simulink model "FCS_MPC_3Phase_SPMSM_TEST1"  (R2022a)
settings: Solver=ode23t  StartTime=0.0  StopTime=0.2  RelTol=1e-3  AbsTol=1e-3  EnableMultiTasking=on
values from neighbouring files (symbols this model uses):
  f_c = 100000    [FCS_MPC_3Phase_SPMSM_Params.m]
  Ld = 0.0003    [FCS_MPC_3Phase_SPMSM_Params.m]
  Lq = 0.0003    [FCS_MPC_3Phase_SPMSM_Params.m]
  np = 4    [FCS_MPC_3Phase_SPMSM_Params.m]
  psiPM = 0.0075    [FCS_MPC_3Phase_SPMSM_Params.m]
  R = 0.085    [FCS_MPC_3Phase_SPMSM_Params.m]
  T_50MHz = 1/f_50MHz    (= 2e-08)    [FCS_MPC_3Phase_SPMSM_Params.m]
  u_dc = 24    [FCS_MPC_3Phase_SPMSM_Params.m]
libraries: ee_lib x22, nesl_utility x22, fl_lib x21, simulink x7
(part 1 of 2)
settings Model: Creator=Michael Hoerner  LastModifiedBy=Andre Merx
settings SolverCC: AutoScaleAbsTol=off  AlgebraicLoopSolver=TrustRegion  DecoupledContinuousIntegration=on  MinimalZcImpactIntegration=on
settings DataIOCC: LimitDataPoints=on  MaxDataPoints=10000  ReturnWorkspaceOutputs=off
settings OptimizationCC: BlockReduction=off  ConditionallyExecuteInputs=off  DefaultParameterBehavior=Inlined  StrengthReduction=on  PassReuseOutputArgsAs=Individual arguments  OptimizeBlockOrder=speed  OptimizationPriority=Speed  OptimizationCustomize=off  MultiThreadedLoops=on  EfficientTunableParamExpr=on
settings DebuggingCC: AlgebraicLoopMsg=error  ParameterTunabilityLossMsg=error  UnconnectedInputMsg=warning  UnconnectedOutputMsg=warning  UnconnectedLineMsg=warning  AllowSymbolicDim=off  SFUnexpectedBacktrackingDiag=warning  SFNoUnconditionalDefaultTransitionDiag=warning  SFExecutionAtInitializationDiag=none  SFMachineParentedDataDiag=warning  ArithmeticOperatorsInVariantConditions=warning
settings HardwareCC: ProdBitPerPointer=32  ProdBitPerSizeT=32  ProdBitPerPtrDiffT=32  ProdLargestAtomicFloat=None  ProdIntDivRoundTo=Undefined  ProdEndianess=Unspecified  ProdWordSize=32  ProdHWDeviceType=ASIC/FPGA->ASIC/FPGA  TargetBitPerPointer=64  TargetBitPerSizeT=64  TargetBitPerPtrDiffT=64  TargetLongLongMode=on  TargetIntDivRoundTo=Zero  TargetEndianess=LittleEndian  TargetWordSize=64  TargetHWDeviceType=Custom Processor->MATLAB Host Computer  ProdEqTarget=off
settings SFSimCC: SimUseLocalCustomCode=off  MATLABDynamicMemAlloc=off  CustomCodeUndefinedFunction=UseInterfaceOnly
settings RTWCC: SystemTargetFile=ert.tlc  TemplateMakefile=ert_default_tmf  GenerateReport=on  RTWUseLocalCustomCode=off  IncludeHyperlinkInReport=on  LaunchReport=on  GenerateTraceInfo=on  GenerateTraceReport=on  GenerateTraceReportSl=on  GenerateTraceReportSf=on  GenerateTraceReportEml=on  DLArmComputeVersion=19.05
settings CodeAppCC: ForceParamTrailComments=on  IgnoreCustomStorageClasses=off  OperatorAnnotations=on  SimulinkDataObjDesc=on  SFDataObjDesc=on  InsertBlockDesc=on
settings ERTTargetCC: CodeReplacementLibrary=TI C28x with C99 extensions  GenerateSampleERTMain=on  CodeInterfacePackaging=Reusable function  MultiInstanceErrorCode=Warning  ERTCustomFileTemplate=example_file_process.tlc  ERTFilePackagingFormat=Compact
settings ConfigComp: CovMetricSettings=dw  CovSaveCumulativeToWorkspaceVar=on  CovSaveSingleToWorkspaceVar=on  CovExternalEMLEnable=off  CovSFcnEnable=off
settings SimscapeCC: SimscapeLogDataHistory=10000

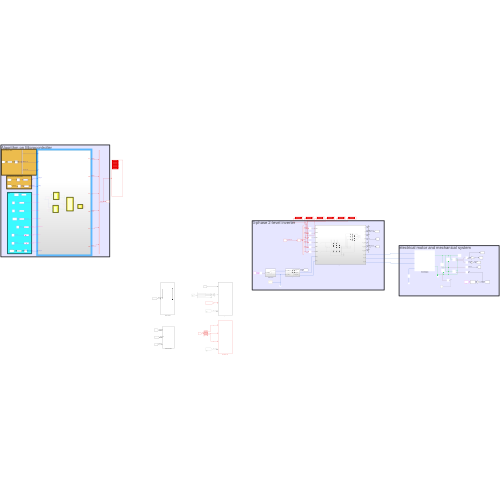
[thumbnail: Simulink's stored preview of the top-level diagram]
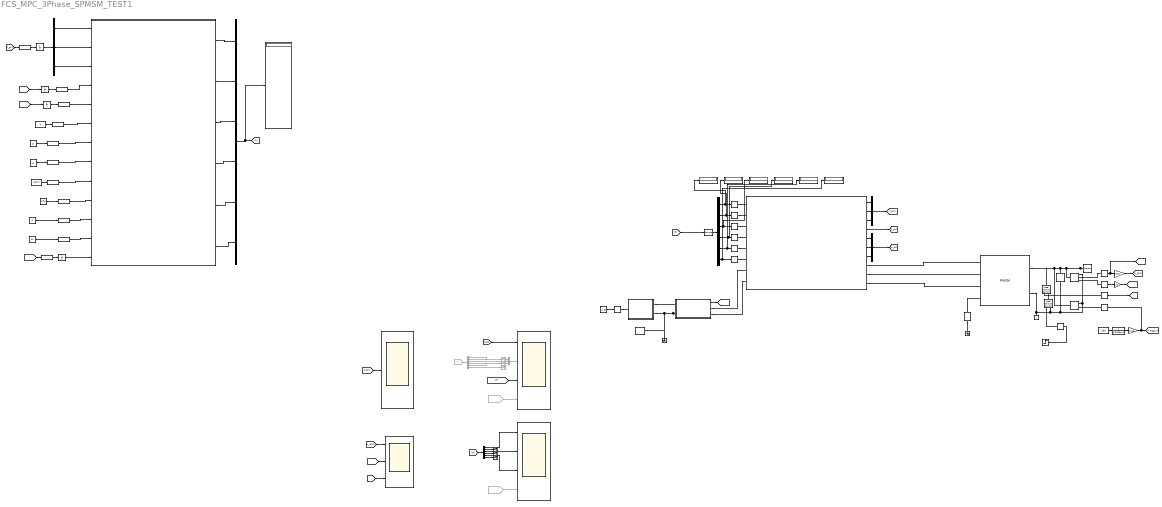
== system FCS_MPC_3Phase_SPMSM_TEST1 ==
  note: electrical motor and mechanical system
  note: 3-phase 2-level inverter
  note: Algorithm on Microcontroller
  note: AXI
  note: Von IP-Core IncreEncoder
  note: Von IP-Core ADC
  3ph_Inverter : Subsystem
  Constant : Constant  Value=Ld
  Constant1 : Constant  Value=R
  Constant11 : Constant  Value=1/f_c
  Constant6 : Constant  Value=u_dc
  Constant8 : Constant  Value=psiPM
  Constant9 : Constant  Value=Lq
  DC_link : Subsystem
  Data Type Conversion : DataTypeConversion  OutDataTypeStr=double  SaturateOnIntegerOverflow=off  RndMeth=Floor
  Data Type Conversion{4,6,10..11} (4 alike) : DataTypeConversion  OutDataTypeStr=fixdt(1,24,20)  SaturateOnIntegerOverflow=off  RndMeth=Floor
  Data Type Conversion{2,5,7..9,24} (6 alike) : DataTypeConversion  OutDataTypeStr=fixdt(1,18,11)  SaturateOnIntegerOverflow=off  RndMeth=Floor
  Data Type Conversion3 : DataTypeConversion  OutDataTypeStr=fixdt(1,24,11)  SaturateOnIntegerOverflow=off  RndMeth=Floor
  Demux : Demux  Outputs=3
  Demux2 : Demux  Outputs=6
  Demux3 : Demux  Commented=on  Outputs=6
  Demux4 : Demux  Outputs=6
  Display{1..7} (7 alike) : Display
  Electrical Reference1 : fl_lib/Electrical/Electrical Elements/Electrical Reference
      settings: SourceProductBaseCode=PW,SS,VE
  Electrical Reference2 : fl_lib/Electrical/Electrical Elements/Electrical Reference
      settings: SourceProductBaseCode=PW,SS,VE
  From5 : From  Commented=on  GotoTag=T
  From6 : From  Commented=on  GotoTag=PWM_counter
  From8 : From  Commented=on  GotoTag=PWM_counter
  Gain : Gain  Gain=30/pi
  Gain7 : Gain  Gain=np
  Gain8 : Gain  Gain=pi/30
  Ideal Angular Velocity Source1 : fl_lib/Mechanical/Mechanical Sources/Ideal Angular Velocity Source
      settings: SourceProductBaseCode=PW,SS,VE
  Ideal Rotational Motion Sensor1 : fl_lib/Mechanical/Mechanical Sensors/Ideal Rotational Motion Sensor  wrap_angle=simscape.enum.onoff.off  offset=0 deg
      settings: SourceProductBaseCode=PW,SS,VE
  Ideal Torque Sensor : fl_lib/Mechanical/Mechanical Sensors/Ideal Torque Sensor
      settings: SourceProductBaseCode=PW,SS,VE
  Ideal Torque Source : fl_lib/Mechanical/Mechanical Sources/Ideal Torque Source
      settings: SourceProductBaseCode=PW,SS,VE
  Inertia1 : fl_lib/Mechanical/Rotational Elements/Inertia  inertia=J kg*m^2  num_ports=foundation.enum.numPorts2.one  w_specify=off  w_priority=High  w=0 rad/s  w_nominal_specify=off  w_nominal_unit=rad/s  w_nominal_value=1  t_specify=off  t_priority=None  t=0 N*m  t_nominal_specify=off  t_nominal_unit=N*m  t_nominal_value=1
      settings: SourceProductBaseCode=PW,SS,VE
  Mechanical Rotational Reference1 : fl_lib/Mechanical/Rotational Elements/Mechanical Rotational Reference
      settings: SourceProductBaseCode=PW,SS,VE
  Microcontroller Software : Subsystem
  Mux : Mux  Inputs=6
  Mux2 : Mux  Inputs=3
  Mux3 : Mux  Inputs=3
  Mux4 : Mux  Commented=on  Inputs=3
  PS-Simulink Converter6 : nesl_utility/PS-Simulink Converter  PhysicalDomain=network_engine_domain  SubClassName=ps_output  LeftPortType=input  RightPortType=output  PseudoPeriodic=off  Frequencies=[]  VectorFormat=1-D array  Unit=1  AffineConversion=off
      settings: SourceProductBaseCode=SS,PW,VE
  PS-Simulink Converter7 : nesl_utility/PS-Simulink Converter  PhysicalDomain=network_engine_domain  SubClassName=ps_output  LeftPortType=input  RightPortType=output  PseudoPeriodic=off  Frequencies=[]  VectorFormat=1-D array  Unit=1  AffineConversion=off
      settings: SourceProductBaseCode=SS,PW,VE
  PS-Simulink Converter8 : nesl_utility/PS-Simulink Converter  PhysicalDomain=network_engine_domain  SubClassName=ps_output  LeftPortType=input  RightPortType=output  PseudoPeriodic=off  Frequencies=[]  VectorFormat=1-D array  Unit=1  AffineConversion=off
      settings: SourceProductBaseCode=SS,PW,VE
  Permanent Magnet Synchronous Motor1 : ee_lib/Electromechanical/Permanent Magnet/PMSM  port_option=ee.enum.threePhasePort.expanded  winding_type=ee.enum.statorconnection.wye  machine_param=ee.enum.pmsm.parameterization.constant  nPolePairs=np  pmflux_param=1  pm_flux_linkage=psiPM Wb  torque_constant=0.18 N*m/A  back_emf_constant=0.18 V/(rad/s)  stator_param=1  Ld=Ld H  Lq=Lq H  idVec=[-200, 0, 200] A  iqVec=[-200, 0, 200] A  LdMatrix=0.0002 * ones(3, 3) H  LqMatrix=0.0002 * ones(3, 3) H  PmMatrix=0.1 * ones(3, 3) Wb  ktMatrix=0.18 * ones(3, 3) N*m/A  keMatrix=0.18 * ones(3, 3) V/(rad/s)  L0=0.00016 H  Ls=0.0002 H  Lm=-0.00002 H  Ms=0.00002 H  Rs=R Ohm  zero_sequence=ee.enum.park.zerosequence.include  axes_param=2  loss_param=ee.enum.ironloss.none  losses_oc=[0, 0, 0] W  losses_sc=[0, 0, 0] W  f_losses=60 Hz  Isc_losses=95 A  J=0.0 kg*m^2  lam=0 N*m/(rad/s)  i_d_specify=off  i_d_priority=None  i_d=0 A  i_d_nominal_specify=off  i_d_nominal_unit=A  i_d_nominal_value=1  i_q_specify=off  i_q_priority=None  i_q=0 A  i_q_nominal_specify=off  i_q_nominal_unit=A  i_q_nominal_value=1  torque_specify=off  torque_priority=None  torque=0 N*m  torque_nominal_specify=off  torque_nominal_unit=N*m  torque_nominal_value=1  angular_velocity_specify=off  angular_velocity_priority=High  angular_velocity=0 deg/s  angular_velocity_nominal_specify=off  angular_velocity_nominal_unit=rpm  angular_velocity_nominal_value=1  angular_position_specify=off  angular_position_priority=High  angular_position=0 deg  angular_position_nominal_specify=off  angular_position_nominal_unit=deg  angular_position_nominal_value=1  alpha=3.93e-3 1/K  alpha_flux=-0.001 1/K  Tmeas=298.15 K  stator_thermal_mass=100 J/K  rotor_thermal_mass=200 J/K  Rm_percent_rotor=90  Rd_percent_rotor=30  temperatureA_specify=off  temperatureA_priority=High  temperatureA=25 degC  temperatureA_nominal_specify=off  temperatureA_nominal_unit=degC  temperatureA_nominal_value=1  temperatureB_specify=off  temperatureB_priority=High  temperatureB=25 degC  temperatureB_nominal_specify=off  temperatureB_nominal_unit=degC  temperatureB_nominal_value=1  temperatureC_specify=off  temperatureC_priority=High  temperatureC=25 degC  temperatureC_nominal_specify=off  temperatureC_nominal_unit=degC  temperatureC_nominal_value=1  temperatureR_specify=off  temperatureR_priority=High  temperatureR=25 degC  temperatureR_nominal_specify=off  temperatureR_nominal_unit=degC  temperatureR_nominal_value=1
      settings: InternalSimscapePortConfiguration="{\"Bottom\":[],\"Left\":[{\"id\":\"a\",\"label\":\"a\",\"type\":\"foundation.electrical.electrical\"},{\"id\":\"b\",\"label\":\"b\",\"type\":\"foundation.electrical.electrical\"},{\"id\":\"c\",\"label\":\"c\",\"type\":\"foundation.electrical.electrical\"},{\"id\":\"n\",\"label\":\"n\",\"type\":\"foundation.electrical.electrical\"}],\"Right\":[{\"id\":\"R\",\"label\":\"R\",\"type\":\"foundation.mechanical.rotational.rotational\"},{\"id\":\"C\",\"label\":\"C\",\"type\":\"foundation.mechanical.rotational.rotational\"}],\"Top\":[]}"
  Power_Source : Subsystem
  Resistor : fl_lib/Electrical/Electrical Elements/Resistor  R=2e6 Ohm  i_specify=off  i_priority=None  i=0 A  i_nominal_specify=off  i_nominal_unit=A  i_nominal_value=1  v_specify=off  v_priority=None  v=0 V  v_nominal_specify=off  v_nominal_unit=V  v_nominal_value=1
      settings: SourceProductBaseCode=PW,SS,VE
  Rotational Friction : fl_lib/Mechanical/Rotational Elements/Rotational Friction  brkwy_trq=0.0622476 N*m  brkwy_vel=0.1 rad/s  Col_trq=0.03460117 N*m  visc_coef=0.00026373 N*m/(rad/s)  w_specify=off  w_priority=None  w=0 rad/s  w_nominal_specify=off  w_nominal_unit=rad/s  w_nominal_value=1  t_specify=off  t_priority=None  t=0 N*m  t_nominal_specify=off  t_nominal_unit=N*m  t_nominal_value=1
      settings: SourceProductBaseCode=PW,SS,VE
  Simulink-PS Converter{,8..9,13..16} (7 alike) : nesl_utility/Simulink-PS Converter  PhysicalDomain=network_engine_domain  SubClassName=ps_input  LeftPortType=input  RightPortType=output  PseudoPeriodic=off  Frequencies=[]  NoiseDistribution=none  NoiseParameters=[]  Unit=1  AffineConversion=off  FilteringAndDerivatives=provide  SimscapeFilterOrder=1  InputFilterTimeConstant=0.001  UdotUserProvided=0
      settings: SourceProductBaseCode=SS,PW,VE
  Simulink-PS Converter1 : nesl_utility/Simulink-PS Converter  PhysicalDomain=network_engine_domain  SubClassName=ps_input  LeftPortType=input  RightPortType=output  PseudoPeriodic=off  Frequencies=[]  NoiseDistribution=none  NoiseParameters=[]  Unit=1  AffineConversion=off  FilteringAndDerivatives=filter  SimscapeFilterOrder=1  InputFilterTimeConstant=0.001  UdotUserProvided=0
      settings: SourceProductBaseCode=SS,PW,VE
  Simulink-PS Converter10 : nesl_utility/Simulink-PS Converter  PhysicalDomain=network_engine_domain  SubClassName=ps_input  LeftPortType=input  RightPortType=output  PseudoPeriodic=off  Frequencies=[]  NoiseDistribution=none  NoiseParameters=[]  Unit=1  AffineConversion=off  FilteringAndDerivatives=filter  SimscapeFilterOrder=1  InputFilterTimeConstant=0.001  UdotUserProvided=0
      settings: SourceProductBaseCode=SS,PW,VE
  Solver Configuration1 : nesl_utility/Solver Configuration  PhysicalDomain=network_engine_domain  SubClassName=solver  LeftPortType=input  RightPortType=generic  Tones=[]  Harmonics=[]  SimulateNoise=off  Profile=off  UseLocalSampling=off  EnableSwitchedLinearOptims=on  FrequencyDomain=off  UseCCode=off  RelTol=0.001  AbsTol=1e-06  MinStep=1e-09  ToWorkspace=off  RevertToSquareIcSolve=off  NumHomotopyIterations=100  PhasorMode=off  PhasorModeNumHarmonics=1  IndexReductionMethod=DerivativeReplacement  DoDC=off  ResidualTolerance=1e-09  UseLocalSolver=off  LocalSolverChoice=NE_BACKWARD_EULER_ADVANCER  LocalSolverSampleTime=1e-6  DoFixedCost=off  MaxNonlinIter=3  MaxModeIter=2  ComputeImpulses=off  ImpulseIterations=2  LinearAlgebra=Sparse  LinearAlgebraNumThread=0  EquationFormulation=NE_TIME_EF  DelaysMemoryBudget=1024  AutomaticFiltering=on  FilteringTimeConstant=0.001  PartitionStorageMethod=AS_NEEDED  PartitionMemoryBudget=1024  PartitionMethod=FAST
      settings: SourceProductBaseCode=SS,PW,VE
  Step1 : Step  Time=0.08  After=-0.5  SampleTime=0
  Terminator : Terminator  Commented=on
  Terminator1 : Terminator  Commented=on
  Terminator2 : Terminator
  Terminator3 : Terminator  Commented=on
  Terminator4 : Terminator
  Terminator5 : Terminator
  Transfer Fcn : TransferFcn  Denominator=[0.0005 1]
  Unit Delay{3..6} (4 alike) : UnitDelay  SampleTime=1/f_c  HasFrameUpgradeWarning=on
  i_dc : Scope  NumInputPorts=4
  id_ref : Constant  Value=0
  iq_ref : Constant  Value=30
  mechanical values : Scope  NumInputPorts=3
  n_ref : Constant  Value=500
  phase_currents : Scope
  sw_pattern_svm : Scope  NumInputPorts=4
  wires:
  DC_link/1(u_dc_link_measured) -> [u_dc_link]
  Constant6/1 -> Simulink-PS Converter/1
  3ph_Inverter/3(i_3) -> Mux2/3  "i_c"
  3ph_Inverter/2(i_2) -> Mux2/2  "i_b"
  Mux2/1 -> [i_ph]  "i_123"
  PS-Simulink Converter7/1 -> Gain7/1  "theta_m"
  Gain7/1 -> [theta_el]  "theta_el"
  Gain8/1 -> Simulink-PS Converter10/1, [omega_m]
  PS-Simulink Converter6/1 -> [omega_m_m], Gain/1  "omega_m"
  PS-Simulink Converter8/1 -> [torque]
  From5/1 -> Demux3/1
  Demux3/1 -> Mux4/1
  Demux3/3 -> Mux4/2
  Demux3/5 -> Mux4/3
  Demux3/2 -> Terminator/1
  Demux3/4 -> Terminator1/1
  From6/1 -> i_dc/4  "PWM_counter"
  3ph_Inverter/1(i_1) -> Mux2/1  "i_a"
  3ph_Inverter/4(i_dc) -> [i_dc]  "i_dc"
  [i_dc] -> i_dc/1
  Demux3/6 -> Terminator3/1
  [T] -> Data Type Conversion/1
  [i_ph] -> phase_currents/1
  Mux4/1 -> i_dc/2  "T"
  n_ref/1 -> Transfer Fcn/1
  Transfer Fcn/1 -> Gain8/1
  [T] -> i_dc/3
  3ph_Inverter/5(u_1_gnd) -> Mux3/1  "i_a"
  Mux3/1 -> [u_ph]  "i_123"
  3ph_Inverter/6(u_2_gnd) -> Mux3/2  "i_b"
  3ph_Inverter/7(u_3_gnd) -> Mux3/3  "i_c"
  Gain/1 -> [n_RPM]
  Step1/1 -> Simulink-PS Converter1/1
  Data Type Conversion/1 -> Demux4/1
  Demux4/1 -> Display1/1, Simulink-PS Converter8/1
  Demux4/2 -> Display2/1, Simulink-PS Converter9/1
  Demux4/3 -> Display3/1, Simulink-PS Converter13/1
  Demux4/4 -> Display5/1, Simulink-PS Converter14/1
  Demux4/5 -> Display4/1, Simulink-PS Converter15/1
  Demux4/6 -> Simulink-PS Converter16/1, Display6/1
  [torque] -> mechanical values/3  "torque"
  [n_RPM] -> mechanical values/1  "n_RPM"
  [theta_el] -> mechanical values/2  "theta_el"
  Demux2/1 -> sw_pattern_svm/1  "T1"
  Demux2/5 -> sw_pattern_svm/3  "T3"
  Demux2/2 -> Terminator2/1
  Demux2/6 -> Terminator5/1
  [T] -> Demux2/1
  Demux2/3 -> sw_pattern_svm/2  "T2"
  Demux2/4 -> Terminator4/1
  From8/1 -> sw_pattern_svm/4  "PWM_counter"
  [u_dc_link] -> Data Type Conversion2/1
  [i_ph] -> Data Type Conversion24/1
  Unit Delay5/1 -> Data Type Conversion3/1
  Data Type Conversion3/1 -> Microcontroller Software/4(omega_m)
  [omega_m_m] -> Unit Delay5/1
  Unit Delay6/1 -> Data Type Conversion4/1
  [theta_el] -> Unit Delay6/1
  Unit Delay4/1 -> Demux/1  "fc"
  Unit Delay3/1 -> Microcontroller Software/13(u_dc_link)
  Data Type Conversion4/1 -> Microcontroller Software/5(theta_el)
  Data Type Conversion5/1 -> Microcontroller Software/6(Rs)
  Data Type Conversion7/1 -> Microcontroller Software/9(psiPM)
  Constant8/1 -> Data Type Conversion7/1
  Constant1/1 -> Data Type Conversion5/1
  id_ref/1 -> Data Type Conversion8/1
  Data Type Conversion9/1 -> Microcontroller Software/12(iq_ref)
  iq_ref/1 -> Data Type Conversion9/1
  Data Type Conversion8/1 -> Microcontroller Software/11(id_ref)
  Mux/1 -> Display7/1, [T]
  Constant9/1 -> Data Type Conversion11/1
  Constant/1 -> Data Type Conversion10/1
  Data Type Conversion11/1 -> Microcontroller Software/8(Lq)
  Data Type Conversion10/1 -> Microcontroller Software/7(Ld)
  Demux/1 -> Microcontroller Software/1(i1)
  Demux/2 -> Microcontroller Software/2(i2)
  Demux/3 -> Microcontroller Software/3(i3)
  Microcontroller Software/6(HB3B) -> Mux/6
  Microcontroller Software/5(HB3T) -> Mux/5
  Microcontroller Software/4(HB2B) -> Mux/4
  Microcontroller Software/3(HB2T) -> Mux/3
  Microcontroller Software/2(HB1B) -> Mux/2
  Microcontroller Software/1(HB1T) -> Mux/1
  Data Type Conversion24/1 -> Unit Delay4/1
  Constant11/1 -> Data Type Conversion6/1
  Data Type Conversion6/1 -> Microcontroller Software/10(SampleTime)
  Data Type Conversion2/1 -> Unit Delay3/1
  connections:
  DC_link/LConn2 -- Power_Source/RConn2 -- Solver Configuration1/RConn1 -- Electrical Reference1/LConn1
  Inertia1/LConn1 -- Ideal Angular Velocity Source1/LConn1 -- Permanent Magnet Synchronous Motor1/RConn1 -- Ideal Torque Sensor/LConn1 -- Rotational Friction/LConn1 -- Ideal Rotational Motion Sensor1/LConn1
  Ideal Rotational Motion Sensor1/RConn1 -- Ideal Angular Velocity Source1/RConn2 -- Rotational Friction/RConn1 -- Permanent Magnet Synchronous Motor1/RConn2 -- Mechanical Rotational Reference1/LConn1 -- Ideal Torque Source/RConn2
  Simulink-PS Converter14/RConn1 -- 3ph_Inverter/LConn4
  Simulink-PS Converter15/RConn1 -- 3ph_Inverter/LConn5
  Simulink-PS Converter16/RConn1 -- 3ph_Inverter/LConn6
  Power_Source/RConn1 -- DC_link/LConn1
  PS-Simulink Converter6/LConn1 -- Ideal Rotational Motion Sensor1/RConn2
  Simulink-PS Converter/RConn1 -- Power_Source/LConn1
  Simulink-PS Converter8/RConn1 -- 3ph_Inverter/LConn1
  Simulink-PS Converter9/RConn1 -- 3ph_Inverter/LConn2
  DC_link/RConn1 -- 3ph_Inverter/LConn7
  Simulink-PS Converter13/RConn1 -- 3ph_Inverter/LConn3
  DC_link/RConn2 -- 3ph_Inverter/LConn8
  PS-Simulink Converter7/LConn1 -- Ideal Rotational Motion Sensor1/RConn3
  3ph_Inverter/RConn1 -- Permanent Magnet Synchronous Motor1/LConn1
  3ph_Inverter/RConn2 -- Permanent Magnet Synchronous Motor1/LConn2
  3ph_Inverter/RConn3 -- Permanent Magnet Synchronous Motor1/LConn3
  Resistor/LConn1 -- Permanent Magnet Synchronous Motor1/LConn4
  Simulink-PS Converter10/RConn1 -- Ideal Angular Velocity Source1/RConn1
  PS-Simulink Converter8/LConn1 -- Ideal Torque Sensor/RConn2
  Resistor/RConn1 -- Electrical Reference2/LConn1
  Simulink-PS Converter1/RConn1 -- Ideal Torque Source/RConn1
  Ideal Torque Source/LConn1 -- Ideal Torque Sensor/RConn1

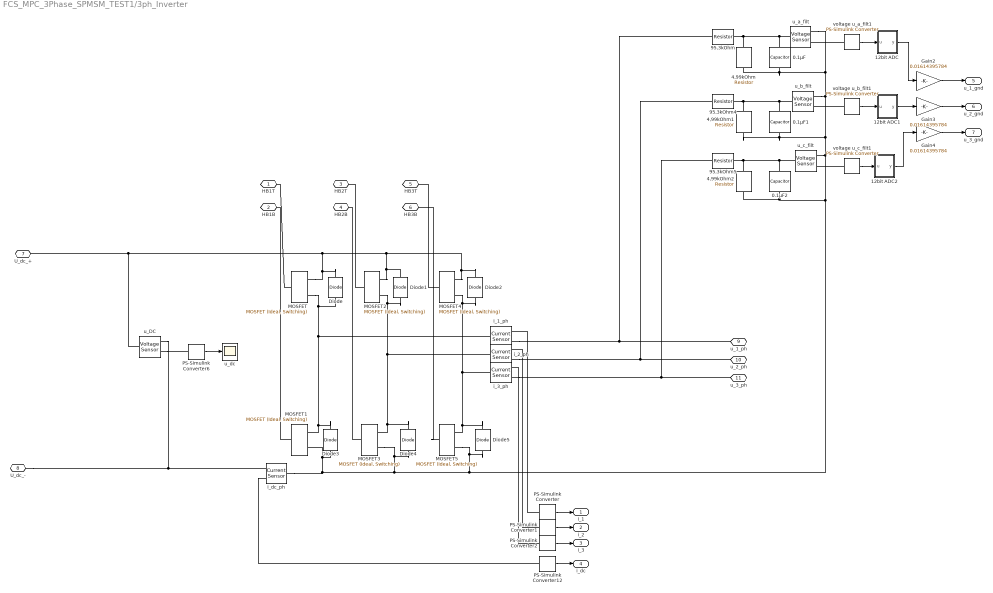
== system FCS_MPC_3Phase_SPMSM_TEST1/3ph_Inverter ==
  0.1µF : ee_lib/Passive/Capacitor  cap_option=0  c=0.1 uF  Cvec=[ 1e-5 1e-6 ] F  Vvec=[ 0 10 ] V  CV_table_symmetry=1  f_vec=[1, 10] kHz  DFext_vec=[.8, 1.2]  enable_C_tol=0  C_tol=5  tol_distribution=1  nSigma=4  r=1e-6 Ohm  g=0 1/Ohm  averaging_period=0 s  enable_operating_limits=0  operating_limit_action=2  max_working_voltage_range=[ -25 25 ] V  power_rating=1 W  enable_faults=0  fault_action=1  Cscale_faulted=100  R_faulted=0.001 Ohm  G_faulted=0 1/Ohm  tau_fault=0.001 s  enable_temporal_fault=0  t_fault=1 s  enable_behavioral_fault=0  max_permissible_voltage_range=[ -100 100 ] V  t_fail_on_voltage=1 s  i_specify=off  i_priority=None  i=0 A  i_nominal_specify=off  i_nominal_unit=A  i_nominal_value=1  v_specify=off  v_priority=None  v=0 V  v_nominal_specify=off  v_nominal_unit=V  v_nominal_value=1  vc_specify=on  vc_priority=High  vc=0 V  vc_nominal_specify=off  vc_nominal_unit=V  vc_nominal_value=1
  0.1µF1 : ee_lib/Passive/Capacitor  cap_option=0  c=0.1 uF  Cvec=[ 1e-5 1e-6 ] F  Vvec=[ 0 10 ] V  CV_table_symmetry=1  f_vec=[1, 10] kHz  DFext_vec=[.8, 1.2]  enable_C_tol=0  C_tol=5  tol_distribution=1  nSigma=4  r=1e-6 Ohm  g=0 1/Ohm  averaging_period=0 s  enable_operating_limits=0  operating_limit_action=2  max_working_voltage_range=[ -25 25 ] V  power_rating=1 W  enable_faults=0  fault_action=1  Cscale_faulted=100  R_faulted=0.001 Ohm  G_faulted=0 1/Ohm  tau_fault=0.001 s  enable_temporal_fault=0  t_fault=1 s  enable_behavioral_fault=0  max_permissible_voltage_range=[ -100 100 ] V  t_fail_on_voltage=1 s  i_specify=off  i_priority=None  i=0 A  i_nominal_specify=off  i_nominal_unit=A  i_nominal_value=1  v_specify=off  v_priority=None  v=0 V  v_nominal_specify=off  v_nominal_unit=V  v_nominal_value=1  vc_specify=on  vc_priority=High  vc=0 V  vc_nominal_specify=off  vc_nominal_unit=V  vc_nominal_value=1
  0.1µF2 : ee_lib/Passive/Capacitor  cap_option=0  c=0.1 uF  Cvec=[ 1e-5 1e-6 ] F  Vvec=[ 0 10 ] V  CV_table_symmetry=1  f_vec=[1, 10] kHz  DFext_vec=[.8, 1.2]  enable_C_tol=0  C_tol=5  tol_distribution=1  nSigma=4  r=1e-6 Ohm  g=0 1/Ohm  averaging_period=0 s  enable_operating_limits=0  operating_limit_action=2  max_working_voltage_range=[ -25 25 ] V  power_rating=1 W  enable_faults=0  fault_action=1  Cscale_faulted=100  R_faulted=0.001 Ohm  G_faulted=0 1/Ohm  tau_fault=0.001 s  enable_temporal_fault=0  t_fault=1 s  enable_behavioral_fault=0  max_permissible_voltage_range=[ -100 100 ] V  t_fail_on_voltage=1 s  i_specify=off  i_priority=None  i=0 A  i_nominal_specify=off  i_nominal_unit=A  i_nominal_value=1  v_specify=off  v_priority=None  v=0 V  v_nominal_specify=off  v_nominal_unit=V  v_nominal_value=1  vc_specify=on  vc_priority=High  vc=0 V  vc_nominal_specify=off  vc_nominal_unit=V  vc_nominal_value=1
  12bit ADC : MATLAB Function  TreatAsAtomicUnit=on
  12bit ADC1 : MATLAB Function  TreatAsAtomicUnit=on
  12bit ADC2 : MATLAB Function  TreatAsAtomicUnit=on
  4,99kOhm : ee_lib/Passive/Resistor  R=4990 Ohm  enable_R_tol=0  R_tol=5  tol_distribution=1  nSigma=4  enable_operating_limits=0  operating_limit_action=2  max_working_voltage=100 V  power_rating=1 W  enable_faults=0  fault_action=1  R_faulted=Inf Ohm  enable_temporal_fault=0  t_fault=1 s  enable_behavioral_fault=0  max_permissible_current=1 A  t_fail_on_current=1 s  noise_mode=0  sample_time=0.001 s  repeatability=1  auto_seed=785646024  user_seed=0  Tdevice=25 degC  power_derating_T1=70 degC  power_derating_T2=155 degC  operating_temperature_range_vec=[-50, 150] degC  alpha=3.93e-3 1/K  Tmeas=25 degC  thermal_mass=100 J/K  temperature_specify=off  temperature_priority=High  temperature=298.15 K  temperature_nominal_specify=off  temperature_nominal_unit=K  temperature_nominal_value=1
  4,99kOhm1 : ee_lib/Passive/Resistor  R=4990 Ohm  enable_R_tol=0  R_tol=5  tol_distribution=1  nSigma=4  enable_operating_limits=0  operating_limit_action=2  max_working_voltage=100 V  power_rating=1 W  enable_faults=0  fault_action=1  R_faulted=Inf Ohm  enable_temporal_fault=0  t_fault=1 s  enable_behavioral_fault=0  max_permissible_current=1 A  t_fail_on_current=1 s  noise_mode=0  sample_time=0.001 s  repeatability=1  auto_seed=1030500139  user_seed=0  Tdevice=25 degC  power_derating_T1=70 degC  power_derating_T2=155 degC  operating_temperature_range_vec=[-50, 150] degC  alpha=3.93e-3 1/K  Tmeas=25 degC  thermal_mass=100 J/K  temperature_specify=off  temperature_priority=High  temperature=298.15 K  temperature_nominal_specify=off  temperature_nominal_unit=K  temperature_nominal_value=1
  4,99kOhm2 : ee_lib/Passive/Resistor  R=4990 Ohm  enable_R_tol=0  R_tol=5  tol_distribution=1  nSigma=4  enable_operating_limits=0  operating_limit_action=2  max_working_voltage=100 V  power_rating=1 W  enable_faults=0  fault_action=1  R_faulted=Inf Ohm  enable_temporal_fault=0  t_fault=1 s  enable_behavioral_fault=0  max_permissible_current=1 A  t_fail_on_current=1 s  noise_mode=0  sample_time=0.001 s  repeatability=1  auto_seed=3807539760  user_seed=0  Tdevice=25 degC  power_derating_T1=70 degC  power_derating_T2=155 degC  operating_temperature_range_vec=[-50, 150] degC  alpha=3.93e-3 1/K  Tmeas=25 degC  thermal_mass=100 J/K  temperature_specify=off  temperature_priority=High  temperature=298.15 K  temperature_nominal_specify=off  temperature_nominal_unit=K  temperature_nominal_value=1
  95,3kOhm : ee_lib/Passive/Resistor  R=95300 Ohm  enable_R_tol=0  R_tol=5  tol_distribution=1  nSigma=4  enable_operating_limits=0  operating_limit_action=2  max_working_voltage=100 V  power_rating=1 W  enable_faults=0  fault_action=1  R_faulted=Inf Ohm  enable_temporal_fault=0  t_fault=1 s  enable_behavioral_fault=0  max_permissible_current=1 A  t_fail_on_current=1 s  noise_mode=0  sample_time=0.001 s  repeatability=1  auto_seed=123154548  user_seed=0  Tdevice=25 degC  power_derating_T1=70 degC  power_derating_T2=155 degC  operating_temperature_range_vec=[-50, 150] degC  alpha=3.93e-3 1/K  Tmeas=25 degC  thermal_mass=100 J/K  temperature_specify=off  temperature_priority=High  temperature=298.15 K  temperature_nominal_specify=off  temperature_nominal_unit=K  temperature_nominal_value=1
  95,3kOhm4 : ee_lib/Passive/Resistor  R=95300 Ohm  enable_R_tol=0  R_tol=5  tol_distribution=1  nSigma=4  enable_operating_limits=0  operating_limit_action=2  max_working_voltage=100 V  power_rating=1 W  enable_faults=0  fault_action=1  R_faulted=Inf Ohm  enable_temporal_fault=0  t_fault=1 s  enable_behavioral_fault=0  max_permissible_current=1 A  t_fail_on_current=1 s  noise_mode=0  sample_time=0.001 s  repeatability=1  auto_seed=2104110442  user_seed=0  Tdevice=25 degC  power_derating_T1=70 degC  power_derating_T2=155 degC  operating_temperature_range_vec=[-50, 150] degC  alpha=3.93e-3 1/K  Tmeas=25 degC  thermal_mass=100 J/K  temperature_specify=off  temperature_priority=High  temperature=298.15 K  temperature_nominal_specify=off  temperature_nominal_unit=K  temperature_nominal_value=1
  95,3kOhm5 : ee_lib/Passive/Resistor  R=95300 Ohm  enable_R_tol=0  R_tol=5  tol_distribution=1  nSigma=4  enable_operating_limits=0  operating_limit_action=2  max_working_voltage=100 V  power_rating=1 W  enable_faults=0  fault_action=1  R_faulted=Inf Ohm  enable_temporal_fault=0  t_fault=1 s  enable_behavioral_fault=0  max_permissible_current=1 A  t_fail_on_current=1 s  noise_mode=0  sample_time=0.001 s  repeatability=1  auto_seed=721241599  user_seed=0  Tdevice=25 degC  power_derating_T1=70 degC  power_derating_T2=155 degC  operating_temperature_range_vec=[-50, 150] degC  alpha=3.93e-3 1/K  Tmeas=25 degC  thermal_mass=100 J/K  temperature_specify=off  temperature_priority=High  temperature=298.15 K  temperature_nominal_specify=off  temperature_nominal_unit=K  temperature_nominal_value=1
  Diode{,1..5} (6 alike) : ee_lib/Semiconductors & Converters/Diode  ModelType=ee.enum.diode.modelType.pwl  TableType=ee.enum.diode.tableType.IfMat  IfMat=[.07, .12, .19, 1.75, 4.24, 7.32, 11.2; .16, .3, .72, 2.14, 4.02, 6.35, 9.12] A  VfMat=[.9, 1.15, 1.25, 1.5, 1.75, 2.17, 2.6, 2.85; .58, .68, .75, 1.1, 1.38, 1.77, 2.27, 2.7] V  TjVec=[25, 125] degC  VfVec=[.5, .7, .9, 1.3, 1.7, 2.1, 2.5] V  IfVec=[.1, .2, .5, 1, 2, 4, 7, 10] A  Vf=0.1 V  Ron=0.001 Ohm  Goff=1e-5 1/Ohm  prmExp=ee.enum.diode.expParam.useTwo  I12=[.0137, .545] A  V12=[.6, .7] V  RS=0 Ohm  Tmeas=25 degC  IS=1e-12 A  ec=1  I1=0.0137 A  V1=0.6 V  N_series=1  N_parallel=1  Rz=0.3 Ohm  BV=inf V  C_param=ee.enum.diode.capParam.fixed  CJ=0 pF  CJ0=5 pF  Vvec=[.1, 10, 100] V  Cvec=[3.5, 1, .4] pF  VJ=1 V  Mgrad=0.5  FC=0.5  Q_param=ee.enum.diode.recoveryParam.off  iRM=-7.15 A  iF=4 A  didt=-750 A/us  trr_factor=3  trr=115 ns  Qrr=150 s*nA  Vr=-600 V  Ls=150 nH  Erec=0.03 J  TT=50 ns  tau=100 ns  T_param=ee.enum.diode.temperatureParam.off  Tdevice=25 degC  I1_T2=0.245 A  V1_T2=0.5 V  IS_T2=1.25e-7 A  Tmeas2=125 degC  XTI_param=ee.enum.diode.xtiParam.pn  XTI=3  EG_param=ee.enum.diode.egapParam.material_si  EG=1.11 eV  dBVdT=0 V/K  enable_faults=simscape.enum.onoff.off  fault_action=simscape.enum.assert.action.none  fault_types=ee.enum.diode.faults.open  tau_fault=1e-3 s  IfMat_faulted=[.07, .12, .19, 1.75, 4.24, 7.32, 11.2; .16, .3, .72, 2.14, 4.02, 6.35, 9.12] A  VfMat_faulted=[.9, 1.15, 1.25, 1.5, 1.75, 2.17, 2.6, 2.85; .58, .68, .75, 1.1, 1.38, 1.77, 2.27, 2.7] V  VfVec_faulted=[.5, .7, .9, 1.3, 1.7, 2.1, 2.5] V  IfVec_faulted=[.1, .2, .5, 1, 2, 4, 7, 10] A  Ropen_faulted=1000 Ohm  Gshort_faulted=1000 1/Ohm  Vf_faulted=0.6 V  Ron_faulted=0.3 Ohm  Goff_faulted=1e-8 S  I12_faulted=[.0137, .545] A  V12_faulted=[.6, .7] V  IS_faulted=1e-12 A  ec_faulted=1  I1_faulted=0.0137 A  V1_faulted=0.6 V  RS_faulted=0 Ohm  Rz_faulted=0.3 Ohm  BV_faulted=inf V  Cscale_faulted=100  enable_temporal_fault=simscape.enum.onoff.off  t_fault=inf s  enable_behavioral_fault=simscape.enum.onoff.off  max_permissible_voltage=inf V  n_fail_on_voltage=1  max_permissible_current=inf A  t_fail_on_current=1 s  max_permissible_dVdt=inf V/s  enable_fault_input=simscape.enum.onoff.off  i_specify=off  i_priority=None  i=0 A  i_nominal_specify=off  i_nominal_unit=A  i_nominal_value=1  v_specify=off  v_priority=None  v=0 V  v_nominal_specify=off  v_nominal_unit=V  v_nominal_value=1  i_diode_specify=off  i_diode_priority=None  i_diode=0 A  i_diode_nominal_specify=off  i_diode_nominal_unit=A  i_diode_nominal_value=1  v_diode_specify=off  v_diode_priority=None  v_diode=0 V  v_diode_nominal_specify=off  v_diode_nominal_unit=V  v_diode_nominal_value=1  i_capacitor_specify=off  i_capacitor_priority=None  i_capacitor=0 A  i_capacitor_nominal_specify=off  i_capacitor_nominal_unit=A  i_capacitor_nominal_value=1  v_capacitor_specify=off  v_capacitor_priority=None  v_capacitor=0 V  v_capacitor_nominal_specify=off  v_capacitor_nominal_unit=V  v_capacitor_nominal_value=1  power_dissipated_specify=off  power_dissipated_priority=None  power_dissipated=0 W  power_dissipated_nominal_specify=off  power_dissipated_nominal_unit=W  power_dissipated_nominal_value=1  max_permissible_temperature=inf K  t_fail_on_temperature=1 s  thermal_network_parameterization=ee.enum.thermalNetworkTopology.junctionCase  Rth=[0, 10] K/W  Rth_Cauer=[1, 3, 10] K/W  Rth_Foster=[4, 6] K/W  thermal_mass_parameterization=ee.enum.thermalNetwork.timeconstant  thermal_mass=[0, 1] J/K  thermal_mass_Cauer=[.1, .3, 1] J/K  thermal_mass_Foster=[1.5, 3] J/K  thermal_time_constant=[0, 10] s  thermal_time_constant_Cauer=[1, 3, 10] s  thermal_time_constant_Foster=[6, 18] s  thermal_mass_initial_temperatures=[25, 25] degC  thermal_mass_initial_temperatures_Cauer=[25, 25, 25] degC  steadyState_Foster=simscape.enum.onoff.on  Tvec_initial_Foster=[25, 25, 25, 25] degC
  Gain2 : Gain  Gain=0.01614395784
  Gain3 : Gain  Gain=0.01614395784
  Gain4 : Gain  Gain=0.01614395784
  MOSFET{,1..5} (6 alike) : ee_lib/Semiconductors & Converters/MOSFET (Ideal, Switching)  Rds=0.040 Ohm  Goff=1e-6 1/Ohm  Vth=0.7 V  diode_param=1  diode_Vf=0.8 V  diode_Ron=0.001 Ohm  diode_Goff=1e-5 1/Ohm  diode_C=5e-8 F  diode_iRM=-235 A  diode_iF=300 A  diode_idot=-50 A/us  diode_trr_param=1  diode_trr_factor=3  diode_trr=15 us  diode_Qrr=1.5e+3 s*uA  thermal_loss_option=ee.enum.converters.thermalLossOption.constantvalues  Von_data=[0, 1.1, 1.3, 1.45, 1.75, 2.25, 2.7; 0, 1, 1.15, 1.35, 1.7, 2.35, 3] V  Tj=[298.15, 398.15] K  Iout_data=[0, 10, 50, 100, 200, 400, 600] A  Eon_data=[0, .29, 1.43, 2.86, 5.71, 13.14, 22.86; 0, .57, 2.63, 5.14, 10.29, 20.57, 30.29] * 1e-3 J  Eoff_data=[0, .21, 1.07, 2.14, 4.29, 9.86, 17.14; 0, .43, 1.97, 3.86, 7.71, 15.43, 22.71] * 1e-3 J  Tj_loss=[298.15, 398.15] K  Iout_data_loss=[0, 10, 50, 100, 200, 400, 600] A  Eon_scalar=22.86e-3 J  Eoff_scalar=17.14e-3 J  Voff=300 V  Iout_scalar=600 A  diodeModelType=ee.enum.converters.diodeModelType.pwl  diodeTableType=ee.enum.diode.tableType.IfMat  diode_IfMat=[.07, .12, .19, 1.75, 4.24, 7.32, 11.2; .16, .3, .72, 2.14, 4.02, 6.35, 9.12] A  diode_VfMat=[.9, 1.15, 1.25, 1.5, 1.75, 2.17, 2.6, 2.85; .58, .68, .75, 1.1, 1.38, 1.77, 2.27, 2.7] V  diode_TjVec=[25, 125] degC  diode_VfVec=[.5, .7, .9, 1.3, 1.7, 2.1, 2.5] V  diode_IfVec=[.1, .2, .5, 1, 2, 4, 7, 10] A  diode_Vr=-600 V  diode_Ls=150 nH  diode_Erec=0.03 J  thermal_network_parameterization=ee.enum.thermalNetworkTopology.external  Rth=[.03, .2] K/W  Rth_Cauer=[.03, .1, .2] K/W  Rth_Foster=[.03, .2] K/W  thermal_mass_parameterization=ee.enum.thermalNetwork.timeconstant  thermal_mass=[3, 25] J/K  thermal_mass_Cauer=[3, 10, 25] J/K  thermal_mass_Foster=[33, 50] J/K  thermal_time_constant=[.1, 5] s  thermal_time_constant_Cauer=[.1, 1, 5] s  thermal_time_constant_Foster=[1, 10] s  thermal_mass_initial_temperatures=[25, 25] degC  thermal_mass_initial_temperatures_Cauer=[25, 25, 25] degC  junction_thermal_mass=0.1 J/K  steadyState_Foster=simscape.enum.onoff.on  Tvec_initial_Foster=[25, 25, 25, 25] degC  no_thermal_network=0  junction_temperature_specify=off  junction_temperature_priority=None  junction_temperature=25 degC  junction_temperature_nominal_specify=off  junction_temperature_nominal_unit=degC  junction_temperature_nominal_value=1  vT_specify=off  vT_priority=None  vT=0 V  vT_nominal_specify=off  vT_nominal_unit=V  vT_nominal_value=1  Qj_specify=off  Qj_priority=None  Qj=0 W  Qj_nominal_specify=off  Qj_nominal_unit=W  Qj_nominal_value=1
  PS-Simulink Converter{,1..2,12} (4 alike) : nesl_utility/PS-Simulink Converter  PhysicalDomain=network_engine_domain  SubClassName=ps_output  LeftPortType=input  RightPortType=output  PseudoPeriodic=off  Frequencies=[]  VectorFormat=1-D array  Unit=A  AffineConversion=off
      settings: SourceProductBaseCode=SS,PW,VE
  PS-Simulink Converter6 : nesl_utility/PS-Simulink Converter  PhysicalDomain=network_engine_domain  SubClassName=ps_output  LeftPortType=input  RightPortType=output  PseudoPeriodic=off  Frequencies=[]  VectorFormat=1-D array  Unit=V  AffineConversion=off
      settings: SourceProductBaseCode=SS,PW,VE
  i_1_ph : fl_lib/Electrical/Electrical Sensors/Current Sensor
      settings: SourceProductBaseCode=PW,SS,VE
  i_2_ph : fl_lib/Electrical/Electrical Sensors/Current Sensor
      settings: SourceProductBaseCode=PW,SS,VE
  i_3_ph : fl_lib/Electrical/Electrical Sensors/Current Sensor
      settings: SourceProductBaseCode=PW,SS,VE
  i_dc_ph : fl_lib/Electrical/Electrical Sensors/Current Sensor
      settings: SourceProductBaseCode=PW,SS,VE
  u_DC : fl_lib/Electrical/Electrical Sensors/Voltage Sensor
      settings: SourceProductBaseCode=PW,SS,VE  LogSimulationData=on
  u_a_filt : fl_lib/Electrical/Electrical Sensors/Voltage Sensor
      settings: SourceProductBaseCode=PW,SS,VE  LogSimulationData=on
  u_b_filt : fl_lib/Electrical/Electrical Sensors/Voltage Sensor
      settings: SourceProductBaseCode=PW,SS,VE  LogSimulationData=on
  u_c_filt : fl_lib/Electrical/Electrical Sensors/Voltage Sensor
      settings: SourceProductBaseCode=PW,SS,VE  LogSimulationData=on
  u_dc : Scope
  voltage u_a_filt1 : nesl_utility/PS-Simulink Converter  PhysicalDomain=network_engine_domain  SubClassName=ps_output  LeftPortType=input  RightPortType=output  PseudoPeriodic=off  Frequencies=[]  VectorFormat=1-D array  Unit=V  AffineConversion=off
      settings: SourceProductBaseCode=SS,PW,VE
  voltage u_b_filt1 : nesl_utility/PS-Simulink Converter  PhysicalDomain=network_engine_domain  SubClassName=ps_output  LeftPortType=input  RightPortType=output  PseudoPeriodic=off  Frequencies=[]  VectorFormat=1-D array  Unit=V  AffineConversion=off
      settings: SourceProductBaseCode=SS,PW,VE
  voltage u_c_filt1 : nesl_utility/PS-Simulink Converter  PhysicalDomain=network_engine_domain  SubClassName=ps_output  LeftPortType=input  RightPortType=output  PseudoPeriodic=off  Frequencies=[]  VectorFormat=1-D array  Unit=V  AffineConversion=off
      settings: SourceProductBaseCode=SS,PW,VE
  HB1T : PMIOPort  Side=Left
  HB1B : PMIOPort  Port=2  Side=Left
  HB2T : PMIOPort  Port=3  Side=Left
  HB2B : PMIOPort  Port=4  Side=Left
  HB3T : PMIOPort  Port=5  Side=Left
  HB3B : PMIOPort  Port=6  Side=Left
  U_dc_+ : PMIOPort  Port=7  Side=Left
  U_dc_- : PMIOPort  Port=8  Side=Left
  u_1_ph : PMIOPort  Port=9  Side=Right
  u_2_ph : PMIOPort  Port=10  Side=Right
  u_3_ph : PMIOPort  Port=11  Side=Right
  i_1 : Outport  VectorParamsAs1DForOutWhenUnconnected=off
  i_2 : Outport  Port=2  VectorParamsAs1DForOutWhenUnconnected=off
  i_3 : Outport  Port=3  VectorParamsAs1DForOutWhenUnconnected=off
  i_dc : Outport  Port=4  VectorParamsAs1DForOutWhenUnconnected=off
  u_1_gnd : Outport  Port=5  VectorParamsAs1DForOutWhenUnconnected=off
  u_2_gnd : Outport  Port=6  VectorParamsAs1DForOutWhenUnconnected=off
  u_3_gnd : Outport  Port=7  VectorParamsAs1DForOutWhenUnconnected=off
  wires:
  PS-Simulink Converter/1 -> i_1/1
  PS-Simulink Converter1/1 -> i_2/1
  PS-Simulink Converter2/1 -> i_3/1
  PS-Simulink Converter12/1 -> i_dc/1
  12bit ADC1/1(y) -> Gain3/1
  voltage u_c_filt1/1 -> 12bit ADC2/1(u)
  Gain4/1 -> u_3_gnd/1
  12bit ADC2/1(y) -> Gain4/1
  12bit ADC/1(y) -> Gain2/1
  Gain2/1 -> u_1_gnd/1
  Gain3/1 -> u_2_gnd/1
  voltage u_b_filt1/1 -> 12bit ADC1/1(u)
  voltage u_a_filt1/1 -> 12bit ADC/1(u)
  PS-Simulink Converter6/1 -> u_dc/1
  connections:
  MOSFET2/RConn2 -- Diode1/LConn1 -- i_2_ph/LConn1 -- Diode4/RConn1 -- MOSFET3/RConn1
  MOSFET/RConn1 -- Diode/RConn1 -- Diode2/RConn1 -- MOSFET4/RConn1 -- Diode1/RConn1 -- MOSFET2/RConn1 -- u_DC/LConn1 -- U_dc_+/RConn1
  MOSFET4/RConn2 -- Diode2/LConn1 -- i_3_ph/LConn1 -- Diode5/RConn1 -- MOSFET5/RConn1
  MOSFET2/LConn1 -- HB2T/RConn1
  MOSFET/LConn1 -- HB1T/RConn1
  MOSFET5/LConn1 -- HB3B/RConn1
  MOSFET1/LConn1 -- HB1B/RConn1
  MOSFET4/LConn1 -- HB3T/RConn1
  MOSFET3/LConn1 -- HB2B/RConn1
  i_1_ph/RConn2 -- 95,3kOhm/LConn1 -- u_1_ph/RConn1
  i_2_ph/RConn2 -- 95,3kOhm4/LConn1 -- u_2_ph/RConn1
  i_3_ph/RConn2 -- 95,3kOhm5/LConn1 -- u_3_ph/RConn1
  PS-Simulink Converter/LConn1 -- i_1_ph/RConn1
  PS-Simulink Converter1/LConn1 -- i_2_ph/RConn1
  PS-Simulink Converter2/LConn1 -- i_3_ph/RConn1
  PS-Simulink Converter12/LConn1 -- i_dc_ph/RConn1
  U_dc_-/RConn1 -- i_dc_ph/RConn2 -- u_DC/RConn2
  95,3kOhm5/RConn1 -- 0.1µF2/LConn1 -- u_c_filt/LConn1 -- 4,99kOhm2/LConn1
  0.1µF1/LConn1 -- u_b_filt/LConn1 -- 4,99kOhm1/LConn1 -- 95,3kOhm4/RConn1
  u_a_filt/LConn1 -- 0.1µF/LConn1 -- 4,99kOhm/LConn1 -- 95,3kOhm/RConn1
  voltage u_c_filt1/LConn1 -- u_c_filt/RConn1
  voltage u_a_filt1/LConn1 -- u_a_filt/RConn1
  voltage u_b_filt1/LConn1 -- u_b_filt/RConn1
  MOSFET5/RConn2 -- Diode5/LConn1 -- 0.1µF2/RConn1 -- 4,99kOhm2/RConn1 -- 4,99kOhm1/RConn1 -- 0.1µF1/RConn1 -- 4,99kOhm/RConn1 -- 0.1µF/RConn1 -- u_a_filt/RConn2 -- u_b_filt/RConn2 -- u_c_filt/RConn2 -- Diode4/LConn1 -- MOSFET3/RConn2 -- Diode3/LConn1 -- MOSFET1/RConn2 -- i_dc_ph/LConn1
  MOSFET/RConn2 -- i_1_ph/LConn1 -- Diode3/RConn1 -- MOSFET1/RConn1 -- Diode/LConn1
  u_DC/RConn1 -- PS-Simulink Converter6/LConn1

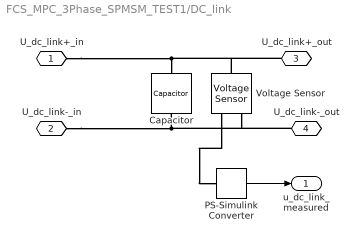
== system FCS_MPC_3Phase_SPMSM_TEST1/DC_link ==
  Capacitor : fl_lib/Electrical/Electrical Elements/Capacitor  c=C_dc_link uF  r=1e-6 Ohm  g=0 1/Ohm  i_specify=off  i_priority=None  i=0 A  i_nominal_specify=off  i_nominal_unit=A  i_nominal_value=1  v_specify=off  v_priority=None  v=0 V  v_nominal_specify=off  v_nominal_unit=V  v_nominal_value=1  vc_specify=off  vc_priority=High  vc=0 V  vc_nominal_specify=off  vc_nominal_unit=V  vc_nominal_value=1
      settings: SourceProductBaseCode=PW,SS,VE
  PS-Simulink Converter : nesl_utility/PS-Simulink Converter  PhysicalDomain=network_engine_domain  SubClassName=ps_output  LeftPortType=input  RightPortType=output  PseudoPeriodic=off  Frequencies=[]  VectorFormat=1-D array  Unit=1  AffineConversion=off
      settings: SourceProductBaseCode=SS,PW,VE
  Voltage Sensor : fl_lib/Electrical/Electrical Sensors/Voltage Sensor
      settings: SourceProductBaseCode=PW,SS,VE
  U_dc_link+_in : PMIOPort  Side=Left
  U_dc_link-_in : PMIOPort  Port=2  Side=Left
  U_dc_link+_out : PMIOPort  Port=3  Side=Right
  U_dc_link-_out : PMIOPort  Port=4  Side=Right
  u_dc_link_measured : Outport  VectorParamsAs1DForOutWhenUnconnected=off
  wires:
  PS-Simulink Converter/1 -> u_dc_link_measured/1
  connections:
  U_dc_link+_in/RConn1 -- Voltage Sensor/LConn1 -- U_dc_link+_out/RConn1 -- Capacitor/LConn1
  U_dc_link-_in/RConn1 -- Voltage Sensor/RConn2 -- U_dc_link-_out/RConn1 -- Capacitor/RConn1
  Voltage Sensor/RConn1 -- PS-Simulink Converter/LConn1

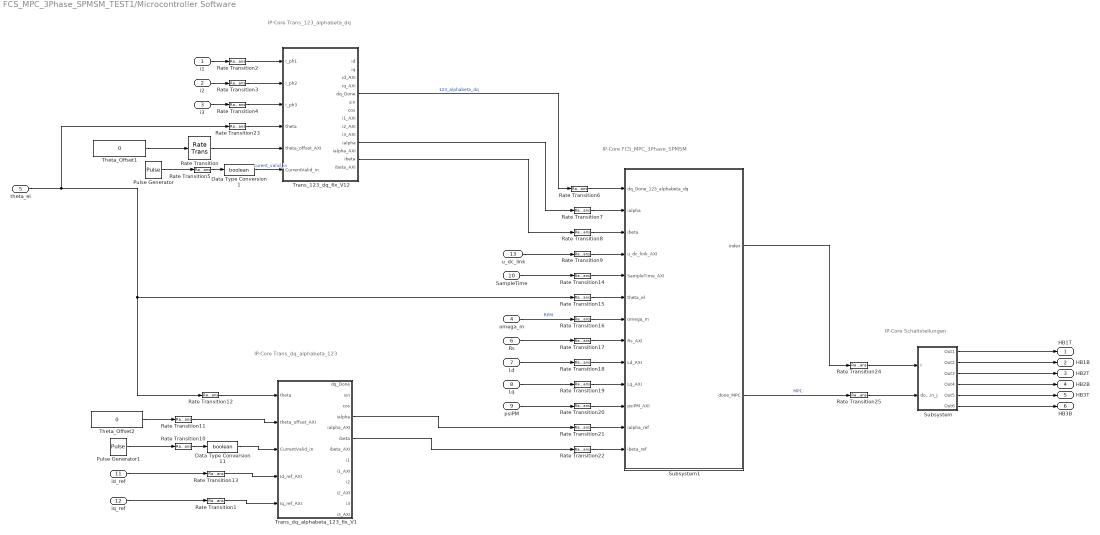
== system FCS_MPC_3Phase_SPMSM_TEST1/Microcontroller Software ==
  note: IP-Core Trans_123_alphabeta_dq
  note: IP-Core Trans_dq_alphabeta_123
  note: IP-Core FCS_MPC_3Phase_SPMSM
  note: IP-Core Schaltstellungen
  i1 : Inport
  i2 : Inport  Port=2
  i3 : Inport  Port=3
  omega_m : Inport  Port=4
  theta_el : Inport  Port=5
  Rs : Inport  Port=6
  Ld : Inport  Port=7
  Lq : Inport  Port=8
  psiPM : Inport  Port=9
  SampleTime : Inport  Port=10
  id_ref : Inport  Port=11
  iq_ref : Inport  Port=12
  u_dc_link : Inport  Port=13
  Data Type Conversion1 : DataTypeConversion  OutDataTypeStr=boolean  SaturateOnIntegerOverflow=off  RndMeth=Floor
  Data Type Conversion11 : DataTypeConversion  OutDataTypeStr=boolean  SaturateOnIntegerOverflow=off  RndMeth=Floor
  Pulse Generator : DiscretePulseGenerator  PulseType=Time based  Period=1/f_c
  Pulse Generator1 : DiscretePulseGenerator  PulseType=Time based  Period=1/f_c  PulseWidth=5
  Rate Transition{,1..5,10..13,23} (11 alike) : RateTransition  OutPortSampleTime=T_50MHz
  Rate Transition{6..9,14..22,24..25} (15 alike) : RateTransition  OutPortSampleTime=T_100MHz
  Subsystem : Subsystem
  Subsystem1 : Subsystem  TreatAsAtomicUnit=on
  Theta_Offset1 : Constant  Value=0  OutDataTypeStr=fixdt(1,24,20)
  Theta_Offset2 : Constant  Value=0  OutDataTypeStr=fixdt(1,24,20)
  Trans_123_dq_fix_V12 : Subsystem  TreatAsAtomicUnit=on
  Trans_dq_alphabeta_123_fix_V1 : Subsystem  TreatAsAtomicUnit=on
  HB1T : Outport
  HB1B : Outport  Port=2
  HB2T : Outport  Port=3
  HB2B : Outport  Port=4
  HB3T : Outport  Port=5
  HB3B : Outport  Port=6
  wires:
  i2/1 -> Rate Transition3/1
  i1/1 -> Rate Transition2/1
  i3/1 -> Rate Transition4/1
  Rate Transition/1 -> Trans_123_dq_fix_V12/5(theta_offset_AXI)
  Theta_Offset1/1 -> Rate Transition/1
  Pulse Generator/1 -> Rate Transition5/1
  Rate Transition5/1 -> Data Type Conversion1/1
  Pulse Generator1/1 -> Rate Transition10/1
  Rate Transition10/1 -> Data Type Conversion11/1
  Theta_Offset2/1 -> Rate Transition11/1
  Rate Transition11/1 -> Trans_dq_alphabeta_123_fix_V1/2(theta_offset_AXI)
  Trans_123_dq_fix_V12/11(ialpha) -> Rate Transition7/1
  Trans_123_dq_fix_V12/13(ibeta) -> Rate Transition8/1
  u_dc_link/1 -> Rate Transition9/1
  omega_m/1 -> Rate Transition16/1  "RPM"
  Rs/1 -> Rate Transition17/1
  Ld/1 -> Rate Transition18/1
  Lq/1 -> Rate Transition19/1
  psiPM/1 -> Rate Transition20/1
  Trans_dq_alphabeta_123_fix_V1/4(ialpha) -> Rate Transition21/1
  Trans_dq_alphabeta_123_fix_V1/6(ibeta) -> Rate Transition22/1
  SampleTime/1 -> Rate Transition14/1
  Subsystem/1(Out1) -> HB1T/1
  Subsystem/2(Out2) -> HB1B/1
  Subsystem/3(Out3) -> HB2T/1
  Subsystem/4(Out4) -> HB2B/1
  Subsystem/5(Out5) -> HB3T/1
  Subsystem/6(Out6) -> HB3B/1
  Trans_123_dq_fix_V12/5(dq_Done) -> Rate Transition6/1  "123_alphabeta_dq"
  Subsystem1/1(Index) -> Rate Transition24/1
  Subsystem1/2(done_MPC) -> Rate Transition25/1  "MPC"
  Data Type Conversion11/1 -> Trans_dq_alphabeta_123_fix_V1/3(CurrentValid_in)
  Data Type Conversion1/1 -> Trans_123_dq_fix_V12/6(CurrentValid_in)  "curent_valid_in"
  id_ref/1 -> Rate Transition13/1
  iq_ref/1 -> Rate Transition1/1
  theta_el/1 -> Rate Transition12/1, Rate Transition15/1, Rate Transition23/1
  Rate Transition12/1 -> Trans_dq_alphabeta_123_fix_V1/1(theta)
  Rate Transition13/1 -> Trans_dq_alphabeta_123_fix_V1/4(Id_ref_AXI)
  Rate Transition1/1 -> Trans_dq_alphabeta_123_fix_V1/5(Iq_ref_AXI)
  Rate Transition2/1 -> Trans_123_dq_fix_V12/1(i_ph1)
  Rate Transition3/1 -> Trans_123_dq_fix_V12/2(i_ph2)
  Rate Transition4/1 -> Trans_123_dq_fix_V12/3(i_ph3)
  Rate Transition6/1 -> Subsystem1/1(dq_Done_123_alphabeta_dq)
  Rate Transition7/1 -> Subsystem1/2(ialpha)
  Rate Transition8/1 -> Subsystem1/3(ibeta)
  Rate Transition9/1 -> Subsystem1/4(u_dc_link_AXI)
  Rate Transition14/1 -> Subsystem1/5(SampleTime_AXI)
  Rate Transition15/1 -> Subsystem1/6(theta_el)
  Rate Transition16/1 -> Subsystem1/7(omega_m)
  Rate Transition17/1 -> Subsystem1/8(Rs_AXI)
  Rate Transition18/1 -> Subsystem1/9(Ld_AXI)
  Rate Transition19/1 -> Subsystem1/10(Lq_AXI)
  Rate Transition20/1 -> Subsystem1/11(psiPM_AXI)
  Rate Transition21/1 -> Subsystem1/12(ialpha_ref)
  Rate Transition22/1 -> Subsystem1/13(ibeta_ref)
  Rate Transition23/1 -> Trans_123_dq_fix_V12/4(theta)
  Rate Transition24/1 -> Subsystem/1(I)
  Rate Transition25/1 -> Subsystem/2(done_min_J)

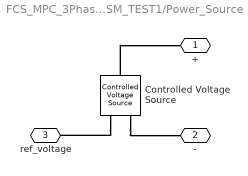
== system FCS_MPC_3Phase_SPMSM_TEST1/Power_Source ==
  Controlled Voltage Source : fl_lib/Electrical/Electrical Sources/Controlled Voltage Source
      settings: SourceProductBaseCode=PW,SS,VE
  + : PMIOPort  Side=Right
  - : PMIOPort  Port=2  Side=Right
  ref_voltage : PMIOPort  Port=3  Side=Left
  connections:
  Controlled Voltage Source/LConn1 -- +/RConn1
  Controlled Voltage Source/RConn2 -- -/RConn1
  Controlled Voltage Source/RConn1 -- ref_voltage/RConn1

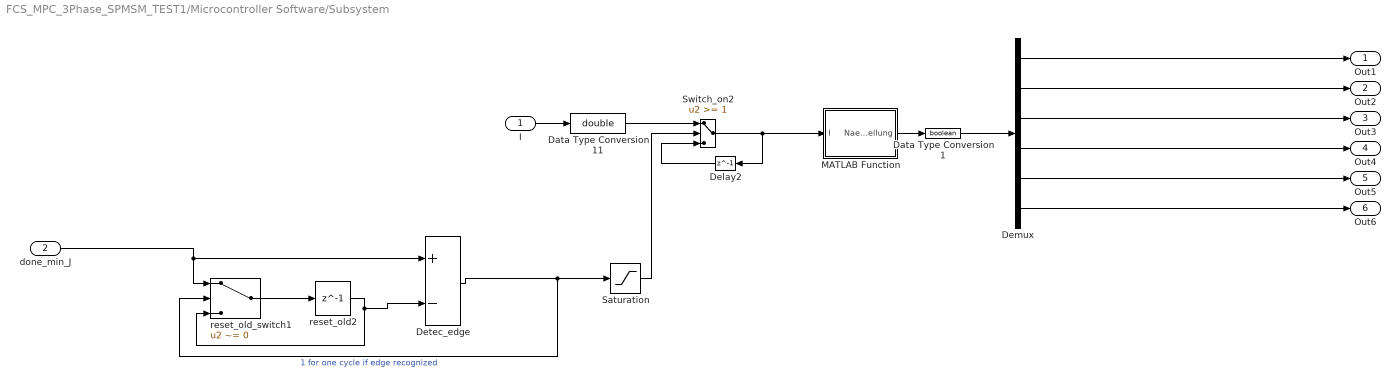
== system FCS_MPC_3Phase_SPMSM_TEST1/Microcontroller Software/Subsystem ==
  I : Inport
  done_min_J : Inport  Port=2
  Data Type Conversion1 : DataTypeConversion  OutDataTypeStr=boolean  SaturateOnIntegerOverflow=off  RndMeth=Floor
  Data Type Conversion11 : DataTypeConversion  OutDataTypeStr=double  SaturateOnIntegerOverflow=off  RndMeth=Floor
  Delay2 : Delay  DelayLength=1
  Demux : Demux  Outputs=6
  Detec_edge : Sum  Inputs=+-  AccumDataTypeStr=int8  OutDataTypeStr=int8
  MATLAB Function : MATLAB Function  TreatAsAtomicUnit=on
  Saturation : Saturate  UpperLimit=1  LowerLimit=0  OutMin=[0]  OutMax=[1]  OutDataTypeStr=fixdt(0,1)
  Switch_on2 : Switch  Threshold=1  OutDataTypeStr=Inherit: Inherit via back propagation  RndMeth=Simplest  SaturateOnIntegerOverflow=off  InputSameDT=off
  reset_old2 : Delay  DelayLength=1
  reset_old_switch1 : Switch  Criteria=u2 ~= 0  SaturateOnIntegerOverflow=off  InputSameDT=off
  Out1 : Outport
  Out2 : Outport  Port=2
  Out3 : Outport  Port=3
  Out4 : Outport  Port=4
  Out5 : Outport  Port=5
  Out6 : Outport  Port=6
  wires:
  Data Type Conversion1/1 -> Demux/1
  Demux/3 -> Out3/1
  MATLAB Function/1(Naechste_Schaltstellung) -> Data Type Conversion1/1
  Demux/4 -> Out4/1
  Demux/1 -> Out1/1
  Demux/2 -> Out2/1
  Demux/6 -> Out6/1
  Demux/5 -> Out5/1
  Switch_on2/1 -> MATLAB Function/1(I), Delay2/1
  Saturation/1 -> Switch_on2/2
  Delay2/1 -> Switch_on2/3
  I/1 -> Data Type Conversion11/1
  done_min_J/1 -> reset_old_switch1/1, Detec_edge/1
  reset_old2/1 -> reset_old_switch1/3, Detec_edge/2
  Detec_edge/1 -> Saturation/1, reset_old_switch1/2  "1 for one cycle if edge recognized"
  reset_old_switch1/1 -> reset_old2/1
  Data Type Conversion11/1 -> Switch_on2/1
